simulink library "INT_EngPrt_TrqLimPTO"  (R2016b)
settings: Solver=VariableStepAuto  StartTime=0.0  StopTime=10.0  RelTol=1e-3
settings Model: Creator=lenovo  LastModifiedBy=lenovo

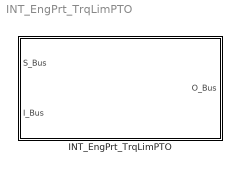
== system INT_EngPrt_TrqLimPTO ==
  INT_EngPrt_TrqLimPTO : Subsystem

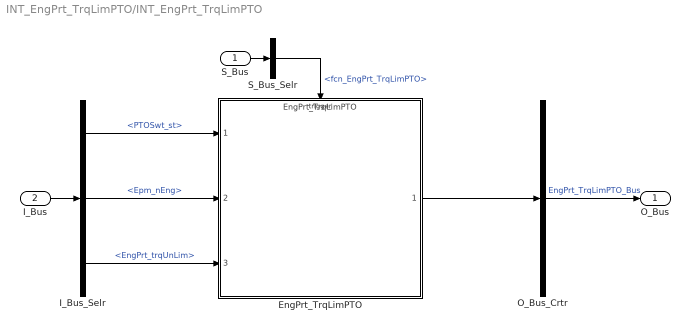
== system INT_EngPrt_TrqLimPTO/INT_EngPrt_TrqLimPTO ==
  S_Bus : Inport
  I_Bus : Inport  Port=2
  EngPrt_TrqLimPTO : ModelReference  ModelNameDialog=EngPrt_TrqLimPTO  SimulationMode=Normal  ModelReferenceVersion=1.11  TriggerPortName=function  TriggerPortTriggerType=function-call  TriggerPortStatesWhenEnabling=held
  I_Bus_Selr : BusSelector  OutputSignals=PTOSwt_st,Epm_nEng,EngPrt_trqUnLim
  O_Bus_Crtr : BusCreator  Inputs=1
  S_Bus_Selr : BusSelector  OutputSignals=fcn_EngPrt_TrqLimPTO
  O_Bus : Outport
  wires:
  S_Bus_Selr/1 -> EngPrt_TrqLimPTO/Trigger  "<fcn_EngPrt_TrqLimPTO>"
  S_Bus/1 -> S_Bus_Selr/1
  I_Bus/1 -> I_Bus_Selr/1
  I_Bus_Selr/1 -> EngPrt_TrqLimPTO/1  "<PTOSwt_st>"
  I_Bus_Selr/2 -> EngPrt_TrqLimPTO/2  "<Epm_nEng>"
  I_Bus_Selr/3 -> EngPrt_TrqLimPTO/3  "<EngPrt_trqUnLim>"
  O_Bus_Crtr/1 -> O_Bus/1  "EngPrt_TrqLimPTO_Bus"
  EngPrt_TrqLimPTO/1 -> O_Bus_Crtr/1
